simulink model "zynqRadioWLAN80211BeaconRxFPGAAD9361AD9364SL"  (R2016a)
settings: Solver=FixedStepDiscrete  SolverMode=SingleTasking  StartTime=0.0  StopTime=inf  RelTol=1e-3
PreLoadFcn:
  | load('commwlan80211BusTypes')
  | openMPDUGUI = true;
PostLoadFcn:
  | zynqRadioWLAN80211BeaconRxFPGAAD9361AD9364SL_params('init')
  | zynqRadioWLAN80211BeaconRxFPGAAD9361AD9364SL_params('scope')
InitFcn:
  | load('commwlan80211BusTypes')
  | openMPDUGUI = true;
  | mpduFigPos= [ 100 100 400 500];
model workspace: external: MAT-File (data not in the file)
undefined symbols (not defined in the file or in its folder): F, p80211, p80211hdl
libraries: simulink x11, hdlsllib x4, commutil2 x3, commwlan80211BeaconLib x2, commdigbbndpm3 x1, commsequence2 x1, commcrc2 x1, dspstat3 x1, dspmlti4 x1, dspsigops x1, dspmathops x1, sdrzblksprivate x1
(part 2 of 2)

== matlab function zynqRadioWLAN80211BeaconRxFPGAAD9361AD9364SL/802.11 WLAN Beacon Frame Receiver/Frame Buffer/data_framer ==
  data: datavld input; data input; RxGo output; p80211 parameter; framed_data output
function [RxGo, framed_data] = dataframer(datavld, data, p80211)
%#codegen

persistent  gooddata_from_prev length_prev_good_data


if isempty(gooddata_from_prev)
    gooddata_from_prev = complex(zeros(128,1));
    length_prev_good_data = 0;
end

if any(datavld) % there is some valid data
    % get the valid data from this frame and append it with the previous
    % stored one, if any
    gooddata_current = data(logical(datavld));
    % append with prev good data
    data_tmp = [gooddata_from_prev(1:length_prev_good_data);gooddata_current];
    if length(data_tmp) > 128
        framed_data = data_tmp(1:128);
        RxGo = 1;
        gooddata_length_athand = length(data_tmp);
        datalen_fornext = gooddata_length_athand -128;
        gooddata_from_prev(1:datalen_fornext) = data_tmp(129:129+datalen_fornext-1);
        length_prev_good_data = datalen_fornext;
    elseif length(data_tmp) == 128 
        framed_data = data_tmp(1:128);
        RxGo = 1;
        gooddata_from_prev =  complex(zeros(128,1));
        length_prev_good_data = 0;
    else % less than 128
        gooddata_length_athand = length(data_tmp);
        datalen_fornext = gooddata_length_athand;      
        gooddata_from_prev(1:gooddata_length_athand) = data_tmp(1:gooddata_length_athand);
        length_prev_good_data = datalen_fornext;
        framed_data = data; % garbage
        RxGo = 0;
    end
    
else % none of the data is valid
    RxGo = 0;
    framed_data = data; %just send the data through
    gooddata_from_prev = complex(zeros(128,1));
    length_prev_good_data = 0;
end
